simulink model "xmc_optical_flow"  (R2019b)
settings: Solver=VariableStepAuto  StartTime=0.0  StopTime=inf  RelTol=1e-3  EnableMultiTasking=on
PostLoadFcn:
  | xmcHubUpdateInstalledDevice(gcs);
model workspace (MAT data in the model file):
  SourceMovingObject = 0
  gainValueHSV = 0.2
undefined symbols (not defined in the file or in its folder): A, AXI4, gray, Kanade, Lucas, N, Rec, SDTV, Stream, xc7vx485tffg1157
libraries: ModelComposer x66, visionconversions x3, visiongeotforms x2, xmcCopyrightNotice x1, visionsinks x1, OpticalFlowRoots x1, visionsources x1, visionutilities x1, dspvision x1
settings Model: Creator=abehbood  LastModifiedBy=abehbood
settings DataIOCC: ReturnWorkspaceOutputs=off
settings OptimizationCC: EfficientMapNaN2IntZero=off  LifeSpan=inf
settings DebuggingCC: SFUnexpectedBacktrackingDiag=warning  SFNoUnconditionalDefaultTransitionDiag=warning  ArithmeticOperatorsInVariantConditions=warning
settings HardwareCC: TargetBitPerLong=64  TargetBitPerPointer=64  TargetBitPerSizeT=64  TargetBitPerPtrDiffT=64  TargetLongLongMode=on  TargetIntDivRoundTo=Zero  TargetEndianess=LittleEndian  TargetWordSize=64  TargetHWDeviceType=MATLAB Host  ProdEqTarget=off
settings SFSimCC: SimUseLocalCustomCode=off  CustomCodeUndefinedFunction=UseInterfaceOnly
settings RTWCC: RTWUseLocalCustomCode=off
settings CodeAppCC: MaxIdLength=128  StateflowObjectComments=on
settings GRTTargetCC: TargetLangStandard=C89/C90 (ANSI)  CombineOutputUpdateFcns=off  GRTInterface=on
settings ConfigComp: CovMetricSettings=dw  CovHtmlReporting=on  CovSaveCumulativeToWorkspaceVar=on  CovSaveSingleToWorkspaceVar=on  CovExternalEMLEnable=off

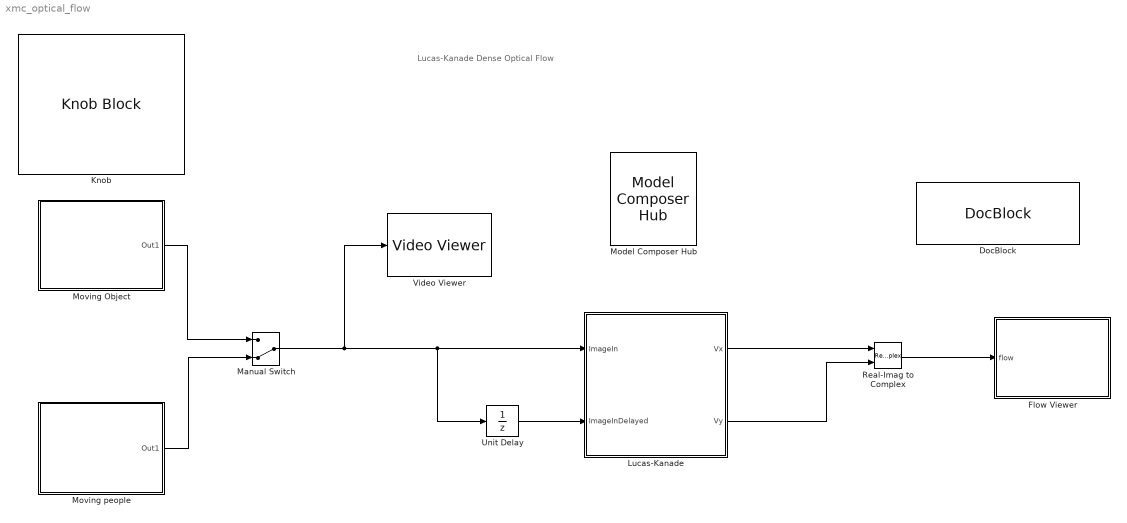
== system xmc_optical_flow ==
  note: Lucas-Kanade Dense Optical Flow
  DocBlock : xmcCopyrightNotice/DocBlock
      content=|
      | (c) Copyright 2017-2018 Xilinx, Inc. All rights reserved.
      |
      | This file contains confidential and proprietary information of Xilinx, Inc.
      | and is protected under U.S. and international copyright and other
      | intellectual property laws.
      |
      | DISCLAIMER
      | This disclaimer is not a license and does not grant any rights to the
      | materials distributed herewith. Except as otherwise provided in a valid
      | license issued to you by Xilinx, and to the maximum extent permitted by
      | applicable law: (1) THESE MATERIALS ARE MADE AVAILABLE "AS IS" AND WITH
      | ALL FAULTS, AND XILINX HEREBY DISCLAIMS ALL WARRANTIES AND CONDITIONS,
      | EXPRESS, IMPLIED, OR STATUTORY, INCLUDING BUT NOT LIMITED TO WARRANTIES
      | OF MERCHANTABILITY, NON-INFRINGEMENT, OR FITNESS FOR ANY PARTICULAR
      | PURPOSE; and (2) Xilinx shall not be liable (whether in contract or tort,
      | including negligence, or under any other theory of liability) for any
      | loss or damage of any kind or nature related to, arising under or in
      | connection with these materials, including for any direct, or any indirect,
      | special, incidental, or consequential loss or damage (including loss of
      | data, profits, goodwill, or any type of loss or damage suffered as a
      | result of any action brought by a third party) even if such damage or loss
      | was reasonably foreseeable or Xilinx had been advised of the possibility
      | of the same.
      |
      | CRITICAL APPLICATIONS
      | Xilinx products are not designed or intended to be fail-safe, or for use
      | in any application requiring fail-safe performance, such as life-support
      | or safety devices or systems, Class III medical devices, nuclear
      | facilities, applications related to the deployment of airbags, or
      | any other applications that could lead to death, personal injury, or
      | severe property or environmental damage (individually and collectively,
      | "Critical Applications"). Customer assumes the sole risk and liability
      | of any use of Xilinx products in Critical Applications, subject only to
      | applicable laws and regulations governing limitations on product liability.
      |
      | THIS COPYRIGHT NOTICE AND DISCLAIMER MUST BE RETAINED AS PART OF
      | THIS FILE AT ALL TIMES.
      settings: SourceProductName=Simulink  SourceProductBaseCode=SL
  Flow Viewer : Subsystem
  Knob : KnobBlock  ScaleMin=-180  ScaleMax=180  TickInterval=45
  Lucas-Kanade : Subsystem  mask{thresh=.0015, d5=[-1 8 0 -8 1]/12, p5=[1 4 6 4 1]/16, b=ones(1,5)/5}
      mask prompts: thresh "Threshold"; d5 "Gradient filter"; p5 "Smoothing filter"; b "Box filter"
      mask init:
      | K  = p5(:)*p5(:)';
  Manual Switch : ManualSwitch  CurrentSetting=0
      settings: OpenFcn=switchCallback(gcb)
  Model Composer Hub : ModelComposer/Model Composer Hub  CodeGeneration=off  SubsystemName=Lucas-Kanade  TargetDirectory=./code  ExportType=HLS C++ code  IpVendor=xilinx.com  IpLibrary=hls  IpVersion=1.0  IpHWLanguage=Verilog  AieCompilerOptions={}  CreateTestbench=off  TestbenchStackSize=10  RunAieSim=off  AieSimTimeout=50000  LaunchVitisAnalyzer=off  RunX86Sim=on  X86SimTimeout=10  ProjDevice=xc7vx485tffg1157-1  ProjDevicePart=xc7vx485tffg1157-1  SamplePeriod=-1  ClockFrequency=300  DataPathParallelism=1
  Moving Object : Subsystem  mask{Angle=98.39185180664066}
      mask prompts: Angle "Angle of motion in degrees:"
  Moving people : Subsystem
  Real-Imag to Complex : RealImagToComplex
  Unit Delay : UnitDelay  SampleTime=-1  HasFrameUpgradeWarning=on
  Video Viewer : VideoViewer  colormapValue=gray(256)  FigPos=[735 508 863 363]
  wires:
  Lucas-Kanade/1(Vx) -> Real-Imag to Complex/1
  Lucas-Kanade/2(Vy) -> Real-Imag to Complex/2
  Unit Delay/1 -> Lucas-Kanade/2(ImageInDelayed)
  Manual Switch/1 -> Unit Delay/1, Lucas-Kanade/1(ImageIn), Video Viewer/1
  Real-Imag to Complex/1 -> Flow Viewer/1(flow)
  Moving Object/1(Out1) -> Manual Switch/1
  Moving people/1(Out1) -> Manual Switch/2

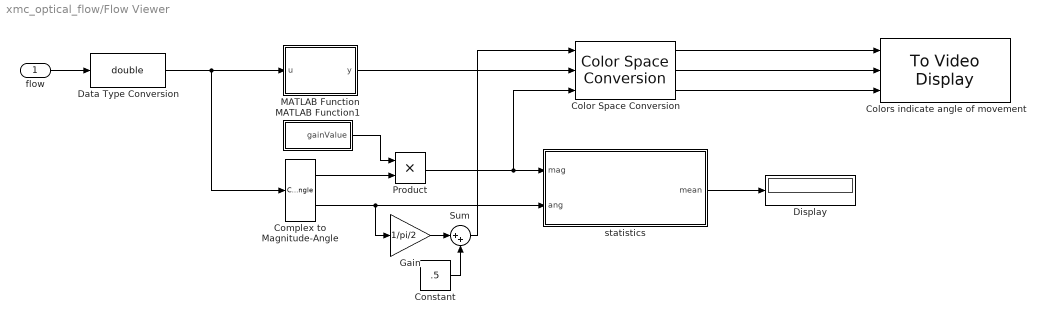
== system xmc_optical_flow/Flow Viewer ==
  flow : Inport
  Color Space Conversion : visionconversions/Color Space  Conversion  conversion=Obsolete  conversionActive=HSV to R'G'B'  wp_str=D65  rec=Rec. 601 (SDTV)  sys=1125/60/2:1  imagePorts=Separate color signals
  Colors indicate angle of movement : visionsinks/To Video Display  windowSizeMode=Normal  openAtMdlStart=on  fullScreen=off  videoWindowX=1226  videoWindowY=338  saveWindowSize=off  videoWindowWidth=670  videoWindowHeight=374  inputColorFormat=RGB  inputType=Obsolete  imagePorts=Separate color signals  OutputDevice=On-screen video monitor  dataOrg=Column-major  isWindowOpen=off
      settings: SourceProductName=Computer Vision Toolbox
  Complex to Magnitude-Angle : ComplexToMagnitudeAngle
  Constant : Constant  Value=.5
  Data Type Conversion : DataTypeConversion  OutDataTypeStr=double
  Display : Display
  Gain : Gain  Gain=1/pi/2  OutDataTypeStr=double
  MATLAB Function : MATLAB Function  TreatAsAtomicUnit=on
  MATLAB Function1 : MATLAB Function  TreatAsAtomicUnit=on
  Product : Product
  Sum : Sum  Inputs=|++
  statistics : MATLAB Function  TreatAsAtomicUnit=on
  wires:
  Color Space Conversion/3 -> Colors indicate angle of movement/3
  Color Space Conversion/2 -> Colors indicate angle of movement/2
  Color Space Conversion/1 -> Colors indicate angle of movement/1
  statistics/1(mean) -> Display/1
  Constant/1 -> Sum/2
  Sum/1 -> Color Space Conversion/1
  Gain/1 -> Sum/1
  Complex to Magnitude-Angle/1 -> Product/2
  MATLAB Function/1(y) -> Color Space Conversion/2
  Complex to Magnitude-Angle/2 -> Gain/1, statistics/2(ang)
  flow/1 -> Data Type Conversion/1
  Data Type Conversion/1 -> MATLAB Function/1(u), Complex to Magnitude-Angle/1
  Product/1 -> Color Space Conversion/3, statistics/1(mag)
  MATLAB Function1/1(gainValue) -> Product/1

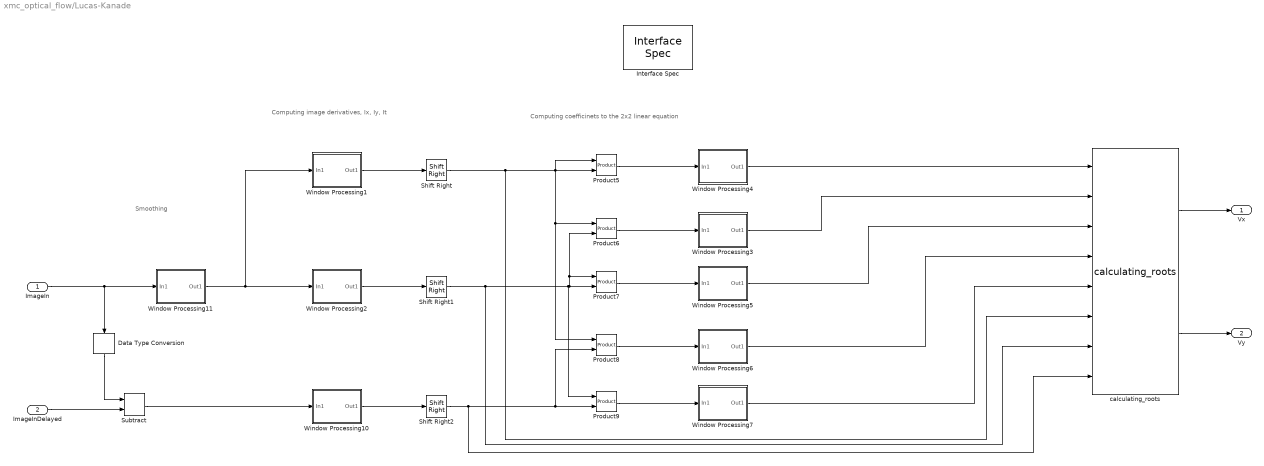
== system xmc_optical_flow/Lucas-Kanade ==
  note: Computing coefficinets to the 2x2
      |  linear equation
  note: Smoothing
  note: Computing image
      | derivatives, Ix, Iy, It
  ImageIn : Inport
  ImageInDelayed : Inport  Port=2
  Data Type Conversion : ModelComposer/Data Type Conversion  OutDataType=fixed  TypeExp=''  Signedness=Unsigned  WordLength=8  FractionalLength=0  RoundingMode=Truncation to minus infinity  OverflowMode=Wrap around
  Interface Spec : ModelComposer/Interface Spec  Return=AXI4-Lite Slave@@  InportInterfaces={'AXI4-Stream@@@N/A@N/A', 'AXI4-Stream@@@N/A@N/A'}  InportHandles={1.300039062500000000e+02, 1.310039062500000000e+02}  InportNames={'ImageIn', 'ImageInDelayed'}  OutportInterfaces={'AXI4-Stream@@@N/A@N/A', 'AXI4-Stream@@@N/A@N/A'}  OutportHandles={3.710037841796875000e+02, 3.720037841796875000e+02}  OutportNames={'Vx', 'Vy'}  Mode=AXI4-Lite Slave  InName1=In1  InMode1=AXI4-Stream  InVFormat1=N/A  InVComponent1=N/A  InName2=In2  InMode2=AXI4-Stream  InVFormat2=N/A  InVComponent2=N/A  InMode3=Default  InVFormat3=N/A  InVComponent3=N/A  InMode4=Default  InVFormat4=N/A  InVComponent4=N/A  InMode5=Default  InVFormat5=N/A  InVComponent5=N/A  InMode6=Default  InVFormat6=N/A  InVComponent6=N/A  InMode7=Default  InVFormat7=N/A  InVComponent7=N/A  InMode8=Default  InVFormat8=N/A  InVComponent8=N/A  OutName1=Out1  OutMode1=AXI4-Stream  OutVFormat1=N/A  OutVComponent1=N/A  OutName2=Out2  OutMode2=AXI4-Stream  OutVFormat2=N/A  OutVComponent2=N/A  OutMode3=Default  OutVFormat3=N/A  OutVComponent3=N/A  OutMode4=Default  OutVFormat4=N/A  OutVComponent4=N/A  OutMode5=Default  OutVFormat5=N/A  OutVComponent5=N/A  OutMode6=Default  OutVFormat6=N/A  OutVComponent6=N/A  OutMode7=Default  OutVFormat7=N/A  OutVComponent7=N/A  OutMode8=Default  OutVFormat8=N/A  OutVComponent8=N/A
  Product{5..9} (5 alike) : ModelComposer/Product
  Shift Right : ModelComposer/Shift Right  ShiftAmount=8
  Shift Right1 : ModelComposer/Shift Right  ShiftAmount=8
  Shift Right2 : ModelComposer/Shift Right  ShiftAmount=8
  Subtract : ModelComposer/Subtract
  Window Processing1 : Subsystem  mask(Window Processing){WindowSize=[1, 5], OutputSize=Same as Input}
      mask prompts: WindowSize "Window Size"; OutputSize "Output Size"
      mask help: Assembles output matrix by applying the kernel subsystem to sub matrices (windows) of the input matrix in row-major order.
      mask init:
      | set_param(gcb, 'LinkStatus', 'inactive');
      mask Help: helpview([xmcGetBlockHTMLPath 'windowprocessing.html']);
      mask TypeOptions WindowSize:
      | Window Processing
      | Master/WindowSize
      mask TypeOptions OutputSize:
      | Window Processing
      | Master/OutputSize
      mask DialogControl Container1 Prompt: Parameters
      mask DialogControl Control5 Prompt: Open Subsystem
      mask DialogControl Control5 Callback:
      | gcb
      | open_system([gcb , '/Kernel'])
      mask Display:
      | xmcDrawBlockIcon();
      | disp('\fontsize{10}   Window \newlineProcessing','texmode','on');
  Window Processing10 : Subsystem  mask(Window Processing){WindowSize=[5, 5], OutputSize=Same as Input}
      mask prompts: WindowSize "Window Size"; OutputSize "Output Size"
      mask help: Assembles output matrix by applying the kernel subsystem to sub matrices (windows) of the input matrix in row-major order.
      mask init:
      | set_param(gcb, 'LinkStatus', 'inactive');
      mask Help: helpview([xmcGetBlockHTMLPath 'windowprocessing.html']);
      mask TypeOptions WindowSize:
      | Window Processing
      | Master/WindowSize
      mask TypeOptions OutputSize:
      | Window Processing
      | Master/OutputSize
      mask DialogControl Container1 Prompt: Parameters
      mask DialogControl Control5 Prompt: Open Subsystem
      mask DialogControl Control5 Callback:
      | gcb
      | open_system([gcb , '/Kernel'])
      mask Display:
      | xmcDrawBlockIcon();
      | disp('\fontsize{10}   Window \newlineProcessing','texmode','on');
  Window Processing11 : Subsystem  mask(Window Processing){WindowSize=[5, 5], OutputSize=Same as Input}
      mask prompts: WindowSize "Window Size"; OutputSize "Output Size"
      mask help: Assembles output matrix by applying the kernel subsystem to sub matrices (windows) of the input matrix in row-major order.
      mask init:
      | set_param(gcb, 'LinkStatus', 'inactive');
      mask Help: helpview([xmcGetBlockHTMLPath 'windowprocessing.html']);
      mask TypeOptions WindowSize:
      | Window Processing
      | Master/WindowSize
      mask TypeOptions OutputSize:
      | Window Processing
      | Master/OutputSize
      mask DialogControl Container1 Prompt: Parameters
      mask DialogControl Control5 Prompt: Open Subsystem
      mask DialogControl Control5 Callback:
      | gcb
      | open_system([gcb , '/Kernel'])
      mask Display:
      | xmcDrawBlockIcon();
      | disp('\fontsize{10}   Window \newlineProcessing','texmode','on');
  Window Processing2 : Subsystem  mask(Window Processing){WindowSize=[5,1], OutputSize=Same as Input}
      mask prompts: WindowSize "Window Size"; OutputSize "Output Size"
      mask help: Assembles output matrix by applying the kernel subsystem to sub matrices (windows) of the input matrix in row-major order.
      mask init:
      | set_param(gcb, 'LinkStatus', 'inactive');
      mask Help: helpview([xmcGetBlockHTMLPath 'windowprocessing.html']);
      mask TypeOptions WindowSize:
      | Window Processing
      | Master/WindowSize
      mask TypeOptions OutputSize:
      | Window Processing
      | Master/OutputSize
      mask DialogControl Container1 Prompt: Parameters
      mask DialogControl Control5 Prompt: Open Subsystem
      mask DialogControl Control5 Callback:
      | gcb
      | open_system([gcb , '/Kernel'])
      mask Display:
      | xmcDrawBlockIcon();
      | disp('\fontsize{10}   Window \newlineProcessing','texmode','on');
  Window Processing3 : Subsystem  mask(Window Processing){WindowSize=[5,5], OutputSize=Same as Input}
      mask prompts: WindowSize "Window Size"; OutputSize "Output Size"
      mask help: Assembles output matrix by applying the kernel subsystem to sub matrices (windows) of the input matrix in row-major order.
      mask init:
      | set_param(gcb, 'LinkStatus', 'inactive');
      mask Help: helpview([xmcGetBlockHTMLPath 'windowprocessing.html']);
      mask TypeOptions WindowSize:
      | Window Processing
      | Master/WindowSize
      mask TypeOptions OutputSize:
      | Window Processing
      | Master/OutputSize
      mask DialogControl Container1 Prompt: Parameters
      mask DialogControl Control5 Prompt: Open Subsystem
      mask DialogControl Control5 Callback:
      | gcb
      | open_system([gcb , '/Kernel'])
      mask Display:
      | xmcDrawBlockIcon();
      | disp('\fontsize{10}   Window \newlineProcessing','texmode','on');
  Window Processing4 : Subsystem  mask(Window Processing){WindowSize=[5,5], OutputSize=Same as Input}
      mask prompts: WindowSize "Window Size"; OutputSize "Output Size"
      mask help: Assembles output matrix by applying the kernel subsystem to sub matrices (windows) of the input matrix in row-major order.
      mask init:
      | set_param(gcb, 'LinkStatus', 'inactive');
      mask Help: helpview([xmcGetBlockHTMLPath 'windowprocessing.html']);
      mask TypeOptions WindowSize:
      | Window Processing
      | Master/WindowSize
      mask TypeOptions OutputSize:
      | Window Processing
      | Master/OutputSize
      mask DialogControl Container1 Prompt: Parameters
      mask DialogControl Control5 Prompt: Open Subsystem
      mask DialogControl Control5 Callback:
      | gcb
      | open_system([gcb , '/Kernel'])
      mask Display:
      | xmcDrawBlockIcon();
      | disp('\fontsize{10}   Window \newlineProcessing','texmode','on');
  Window Processing5 : Subsystem  mask(Window Processing){WindowSize=[5,5], OutputSize=Same as Input}
      mask prompts: WindowSize "Window Size"; OutputSize "Output Size"
      mask help: Assembles output matrix by applying the kernel subsystem to sub matrices (windows) of the input matrix in row-major order.
      mask init:
      | set_param(gcb, 'LinkStatus', 'inactive');
      mask Help: helpview([xmcGetBlockHTMLPath 'windowprocessing.html']);
      mask TypeOptions WindowSize:
      | Window Processing
      | Master/WindowSize
      mask TypeOptions OutputSize:
      | Window Processing
      | Master/OutputSize
      mask DialogControl Container1 Prompt: Parameters
      mask DialogControl Control5 Prompt: Open Subsystem
      mask DialogControl Control5 Callback:
      | gcb
      | open_system([gcb , '/Kernel'])
      mask Display:
      | xmcDrawBlockIcon();
      | disp('\fontsize{10}   Window \newlineProcessing','texmode','on');
  Window Processing6 : Subsystem  mask(Window Processing){WindowSize=[5,5], OutputSize=Same as Input}
      mask prompts: WindowSize "Window Size"; OutputSize "Output Size"
      mask help: Assembles output matrix by applying the kernel subsystem to sub matrices (windows) of the input matrix in row-major order.
      mask init:
      | set_param(gcb, 'LinkStatus', 'inactive');
      mask Help: helpview([xmcGetBlockHTMLPath 'windowprocessing.html']);
      mask TypeOptions WindowSize:
      | Window Processing
      | Master/WindowSize
      mask TypeOptions OutputSize:
      | Window Processing
      | Master/OutputSize
      mask DialogControl Container1 Prompt: Parameters
      mask DialogControl Control5 Prompt: Open Subsystem
      mask DialogControl Control5 Callback:
      | gcb
      | open_system([gcb , '/Kernel'])
      mask Display:
      | xmcDrawBlockIcon();
      | disp('\fontsize{10}   Window \newlineProcessing','texmode','on');
  Window Processing7 : Subsystem  mask(Window Processing){WindowSize=[5,5], OutputSize=Same as Input}
      mask prompts: WindowSize "Window Size"; OutputSize "Output Size"
      mask help: Assembles output matrix by applying the kernel subsystem to sub matrices (windows) of the input matrix in row-major order.
      mask init:
      | set_param(gcb, 'LinkStatus', 'inactive');
      mask Help: helpview([xmcGetBlockHTMLPath 'windowprocessing.html']);
      mask TypeOptions WindowSize:
      | Window Processing
      | Master/WindowSize
      mask TypeOptions OutputSize:
      | Window Processing
      | Master/OutputSize
      mask DialogControl Container1 Prompt: Parameters
      mask DialogControl Control5 Prompt: Open Subsystem
      mask DialogControl Control5 Callback:
      | gcb
      | open_system([gcb , '/Kernel'])
      mask Display:
      | xmcDrawBlockIcon();
      | disp('\fontsize{10}   Window \newlineProcessing','texmode','on');
  calculating_roots : OpticalFlowRoots/calculating_roots  LibraryFunction=calculating_roots  IncludeFiles={'calculating_roots.h'}  SourceFiles={}  IncludeDirectories={}  TemplateParams={' '}  FunctionParamTypes={xmcDataType('void'); xmcDataType('int16_t'); xmcDataType('int16_t'); xmcDataType('int16_t'); xmcDataType('int16_t'); xmcDataType('int16_t'); xmcDataType('int16_t'); xmcDataType('int16_t'); xmcDataType('int16_t'); xmcDataType('float &'); xmcDataType('float &')}  FunctionParamPassbys={0.000000000000000000e+00; 0.000000000000000000e+00; 0.000000000000000000e+00; 0.000000000000000000e+00; 0.000000000000000000e+00; 0.000000000000000000e+00; 0.000000000000000000e+00; 0.000000000000000000e+00; 0.000000000000000000e+00; 1.000000000000000000e+00; 1.000000000000000000e+00}  FunctionParamDimensions={'1'; '1'; '1'; '1'; '1'; '1'; '1'; '1'; '1'; '1'; '1'}  FunctionParamNames={'return'; 'aPix'; 'bPix'; 'cPix'; 'txPix'; 'tyPix'; 'IxPix'; 'IyPix'; 'dtPix'; 'VxPix'; 'VyPix'}  FunctionParamDir={0.000000000000000000e+00; 1.000000000000000000e+00; 1.000000000000000000e+00; 1.000000000000000000e+00; 1.000000000000000000e+00; 1.000000000000000000e+00; 1.000000000000000000e+00; 1.000000000000000000e+00; 1.000000000000000000e+00; 2.000000000000000000e+00; 2.000000000000000000e+00}  FunctionParamSupportsStreaming={false; false; false; false; false; false; false; false; false; false; false}  BufferDepth={'0'}  FunctionParamValues={'0'; '0'; '0'; '0'; '0'; '0'; '0'; '0'; '0'; '0'; '0'}  ThroughputFactors={''}
  Vx : Outport
  Vy : Outport  Port=2
  wires:
  calculating_roots/1 -> Vx/1
  ImageIn/1 -> Data Type Conversion/1, Window Processing11/1(In1)
  Window Processing2/1(Out1) -> Shift Right1/1
  calculating_roots/2 -> Vy/1
  Window Processing10/1(Out1) -> Shift Right2/1
  ImageInDelayed/1 -> Subtract/2
  Window Processing11/1(Out1) -> Window Processing2/1(In1), Window Processing1/1(In1)
  Data Type Conversion/1 -> Subtract/1
  Subtract/1 -> Window Processing10/1(In1)
  Product5/1 -> Window Processing4/1(In1)
  Product6/1 -> Window Processing3/1(In1)
  Product8/1 -> Window Processing6/1(In1)
  Product7/1 -> Window Processing5/1(In1)
  Product9/1 -> Window Processing7/1(In1)
  Shift Right2/1 -> calculating_roots/8, Product9/2, Product8/2
  Window Processing4/1(Out1) -> calculating_roots/1
  Window Processing3/1(Out1) -> calculating_roots/2
  Window Processing5/1(Out1) -> calculating_roots/3
  Window Processing6/1(Out1) -> calculating_roots/4
  Window Processing7/1(Out1) -> calculating_roots/5
  Shift Right/1 -> calculating_roots/6, Product5/1, Product5/2, Product6/1, Product8/1
  Shift Right1/1 -> calculating_roots/7, Product7/2, Product6/2, Product7/1, Product9/1
  Window Processing1/1(Out1) -> Shift Right/1

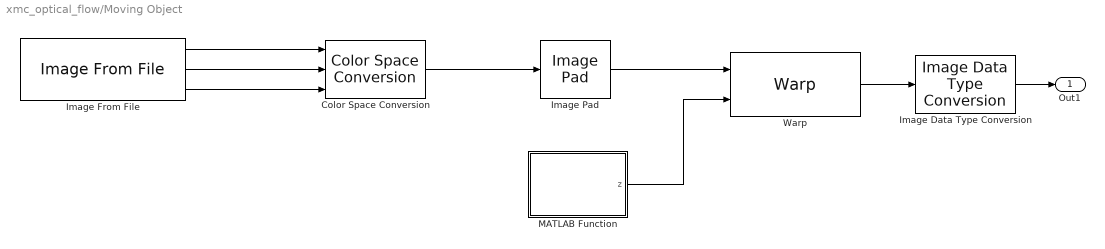
== system xmc_optical_flow/Moving Object ==
  Color Space Conversion : visionconversions/Color Space  Conversion  conversion=Obsolete  conversionActive=R'G'B' to intensity  wp_str=D65  rec=Rec. 601 (SDTV)  sys=1125/60/2:1  imagePorts=Separate color signals
  Image Data Type Conversion : visionconversions/Image Data Type Conversion  outDT=uint8  isSigned=on  wordLen=16  numFracBits=0
      settings: SourceProductName=Computer Vision Toolbox  SourceProductBaseCode=VP
  Image From File : visionsources/Image From File  Tag=vipblks_nd  FileName=object.png  Ts=1  imagePorts=Separate color signals  OutPortLabels=R|G|B  ImageDataType=double  sdImageDataType=uint(8)  Signed=on  WordLength=16  FractionLengthMode=User-defined  FractionLength=15
      settings: SourceProductName=Computer Vision Toolbox
  Image Pad : visionutilities/Image Pad  method=Constant  valSrc=Specify via dialog  value=0  spec=Pad size  rowDirection=Both left and right  outRowsMode=User-specified  rowSize=95  outColSize=10  colDirection=Both top and bottom  outColsMode=User-specified  colSize=95  outRowSize=12  trunc_flag=None
      settings: SourceProductName=Computer Vision Toolbox  SourceProductBaseCode=VP
  MATLAB Function : MATLAB Function  TreatAsAtomicUnit=on
  Warp : visiongeotforms/Warp  TransformMatrixSource=Input port  TransformMatrix=eye( 3 )  InterpolationMethod=Bilinear  BackgroundFillValue=0  OutputImagePositionSource=Same as input image  OutputImagePosition=[ 1, 1, 512, 512 ]  ROIInputPort=off  ROIValidityOutputPort=off  SimulateUsing=Interpreted execution
      settings: SourceProductName=Computer Vision Toolbox  SourceProductBaseCode=VP
  Out1 : Outport
  wires:
  Image Data Type Conversion/1 -> Out1/1
  Color Space Conversion/1 -> Image Pad/1
  Image From File/3 -> Color Space Conversion/3
  Image Pad/1 -> Warp/1
  Image From File/1 -> Color Space Conversion/1
  Image From File/2 -> Color Space Conversion/2
  MATLAB Function/1(z) -> Warp/2
  Warp/1 -> Image Data Type Conversion/1

== system xmc_optical_flow/Moving people ==
  From Multimedia File : dspvision/From Multimedia File  inputFilename=vipmen.avi  readRange=[1 Inf]  loop=on  numPlays=inf  outputStreams=Video only  videoDataType=uint8  audioDataType=int16  inheritSampleTime=off  userDefinedSampleTime=1  noAudioOutput=off  isIntensityVideo=off  fourcc=Intensity  colorVideoFormat=One multidimensional signal  outputEOF=off  dataOrg=Column-major  audioFrameSize=1024  computeAudioFrameSize=off  outSamplingMode=Sample based
      settings: SourceProductName=DSP System Toolbox  SourceProductBaseCode=DS
  Resize : visiongeotforms/Resize  specify=Number of output rows and columns  rfactor=[200 150]  outCols=25  outRows=25  outRowsCols=[200 200]  interp_method=Bilinear  antialias=on  useROI=off  roiFlag=off  roundingMode=Nearest  overflowMode=on  prodOutputMode=Binary point scaling  prodOutputWordLength=32  prodOutputFracLength=10  prodOutputSlope=2^-10  accumSlope=2^-10  outputSlope=2^-10
      settings: SourceProductName=Computer Vision Toolbox  SourceProductBaseCode=VP
  Out1 : Outport
  wires:
  Resize/1 -> Out1/1
  From Multimedia File/1 -> Resize/1

== system xmc_optical_flow/Lucas-Kanade/Window Processing1 ==
  In1 : Inport
  Kernel : Subsystem
  Window Processing Master : ModelComposer/Window Processing Master  Description=Performs multiplication  WindowSize=WindowSize  OutputSize=Same as Input
  Window Processing Slave : ModelComposer/Window Processing Slave  Description=Performs multiplication
  Out1 : Outport
  wires:
  Window Processing Slave/1 -> Window Processing Master/2
  Kernel/1(Out1) -> Window Processing Slave/1
  Window Processing Master/2 -> Kernel/1(In1)
  In1/1 -> Window Processing Master/1
  Window Processing Master/1 -> Out1/1

== system xmc_optical_flow/Lucas-Kanade/Window Processing10 ==
  In1 : Inport
  Kernel : Subsystem
  Window Processing Master : ModelComposer/Window Processing Master  Description=Performs multiplication  WindowSize=WindowSize  OutputSize=Same as Input
  Window Processing Slave : ModelComposer/Window Processing Slave  Description=Performs multiplication
  Out1 : Outport
  wires:
  Window Processing Slave/1 -> Window Processing Master/2
  Kernel/1(Out1) -> Window Processing Slave/1
  Window Processing Master/2 -> Kernel/1(In1)
  In1/1 -> Window Processing Master/1
  Window Processing Master/1 -> Out1/1

== system xmc_optical_flow/Lucas-Kanade/Window Processing11 ==
  In1 : Inport
  Kernel : Subsystem
  Window Processing Master : ModelComposer/Window Processing Master  Description=Performs multiplication  WindowSize=WindowSize  OutputSize=Same as Input
  Window Processing Slave : ModelComposer/Window Processing Slave  Description=Performs multiplication
  Out1 : Outport
  wires:
  Window Processing Master/1 -> Out1/1
  In1/1 -> Window Processing Master/1
  Window Processing Master/2 -> Kernel/1(In1)
  Kernel/1(Out1) -> Window Processing Slave/1
  Window Processing Slave/1 -> Window Processing Master/2

== system xmc_optical_flow/Lucas-Kanade/Window Processing2 ==
  In1 : Inport
  Kernel : Subsystem
  Window Processing Master : ModelComposer/Window Processing Master  Description=Performs multiplication  WindowSize=WindowSize  OutputSize=Same as Input
  Window Processing Slave : ModelComposer/Window Processing Slave  Description=Performs multiplication
  Out1 : Outport
  wires:
  Window Processing Master/1 -> Out1/1
  In1/1 -> Window Processing Master/1
  Window Processing Master/2 -> Kernel/1(In1)
  Kernel/1(Out1) -> Window Processing Slave/1
  Window Processing Slave/1 -> Window Processing Master/2

== system xmc_optical_flow/Lucas-Kanade/Window Processing3 ==
  In1 : Inport
  Kernel : Subsystem
  Window Processing Master : ModelComposer/Window Processing Master  Description=Performs multiplication  WindowSize=WindowSize  OutputSize=Same as Input
  Window Processing Slave : ModelComposer/Window Processing Slave  Description=Performs multiplication
  Out1 : Outport
  wires:
  Window Processing Slave/1 -> Window Processing Master/2
  Kernel/1(Out1) -> Window Processing Slave/1
  Window Processing Master/2 -> Kernel/1(In1)
  In1/1 -> Window Processing Master/1
  Window Processing Master/1 -> Out1/1

== system xmc_optical_flow/Lucas-Kanade/Window Processing4 ==
  In1 : Inport
  Kernel : Subsystem
  Window Processing Master : ModelComposer/Window Processing Master  Description=Performs multiplication  WindowSize=WindowSize  OutputSize=Same as Input
  Window Processing Slave : ModelComposer/Window Processing Slave  Description=Performs multiplication
  Out1 : Outport
  wires:
  Window Processing Master/1 -> Out1/1
  In1/1 -> Window Processing Master/1
  Window Processing Master/2 -> Kernel/1(In1)
  Kernel/1(Out1) -> Window Processing Slave/1
  Window Processing Slave/1 -> Window Processing Master/2

== system xmc_optical_flow/Lucas-Kanade/Window Processing5 ==
  In1 : Inport
  Kernel : Subsystem
  Window Processing Master : ModelComposer/Window Processing Master  Description=Performs multiplication  WindowSize=WindowSize  OutputSize=Same as Input
  Window Processing Slave : ModelComposer/Window Processing Slave  Description=Performs multiplication
  Out1 : Outport
  wires:
  Window Processing Master/1 -> Out1/1
  In1/1 -> Window Processing Master/1
  Window Processing Master/2 -> Kernel/1(In1)
  Kernel/1(Out1) -> Window Processing Slave/1
  Window Processing Slave/1 -> Window Processing Master/2

== system xmc_optical_flow/Lucas-Kanade/Window Processing6 ==
  In1 : Inport
  Kernel : Subsystem
  Window Processing Master : ModelComposer/Window Processing Master  Description=Performs multiplication  WindowSize=WindowSize  OutputSize=Same as Input
  Window Processing Slave : ModelComposer/Window Processing Slave  Description=Performs multiplication
  Out1 : Outport
  wires:
  Window Processing Slave/1 -> Window Processing Master/2
  Kernel/1(Out1) -> Window Processing Slave/1
  Window Processing Master/2 -> Kernel/1(In1)
  In1/1 -> Window Processing Master/1
  Window Processing Master/1 -> Out1/1

== system xmc_optical_flow/Lucas-Kanade/Window Processing7 ==
  In1 : Inport
  Kernel : Subsystem
  Window Processing Master : ModelComposer/Window Processing Master  Description=Performs multiplication  WindowSize=WindowSize  OutputSize=Same as Input
  Window Processing Slave : ModelComposer/Window Processing Slave  Description=Performs multiplication
  Out1 : Outport
  wires:
  Window Processing Master/1 -> Out1/1
  In1/1 -> Window Processing Master/1
  Window Processing Master/2 -> Kernel/1(In1)
  Kernel/1(Out1) -> Window Processing Slave/1
  Window Processing Slave/1 -> Window Processing Master/2

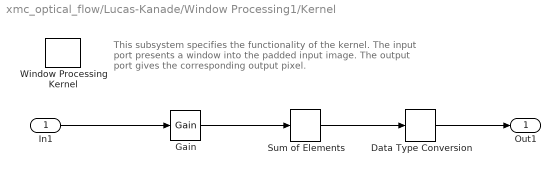
== system xmc_optical_flow/Lucas-Kanade/Window Processing1/Kernel ==
  note: This subsystem specifies the functionality of the kernel.
      | The input port presents a window into the padded input image.
      | The output port gives the corresponding output pixel.
  In1 : Inport
  Data Type Conversion : ModelComposer/Data Type Conversion  OutDataType=int16  TypeExp=''  Signedness=Signed  WordLength=16  FractionalLength=0  RoundingMode=Truncation to minus infinity  OverflowMode=Wrap around
  Gain : ModelComposer/Gain  Gain=fliplr(d5(:)')*256  OutDataType=fixed  TypeExp=''  Signedness=Signed  WordLength=9  FractionalLength=0  RoundingMode=Truncation to minus infinity  OverflowMode=Wrap around  OutputTypeAsInput=off
  Sum of Elements : ModelComposer/Sum of Elements  CollapseDim=2
  Window Processing Kernel : ModelComposer/Window Processing Kernel  Description=Performs multiplication  SubsystemName='optical_flow_moc/Lucas-Kanade/Window Processing1/Kernel'  TargetDirectory='./Kernel'
  Out1 : Outport
  wires:
  In1/1 -> Gain/1
  Gain/1 -> Sum of Elements/1
  Sum of Elements/1 -> Data Type Conversion/1
  Data Type Conversion/1 -> Out1/1

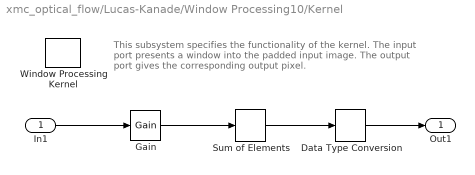
== system xmc_optical_flow/Lucas-Kanade/Window Processing10/Kernel ==
  note: This subsystem specifies the functionality of the kernel.
      | The input port presents a window into the padded input image.
      | The output port gives the corresponding output pixel.
  In1 : Inport
  Data Type Conversion : ModelComposer/Data Type Conversion  OutDataType=int16  TypeExp=''  Signedness=Signed  WordLength=16  FractionalLength=0  RoundingMode=Truncation to minus infinity  OverflowMode=Wrap around
  Gain : ModelComposer/Gain  Gain=p5(:)*p5(:)'*256  OutDataType=uint8  TypeExp=''  Signedness=Unsigned  WordLength=16  FractionalLength=16  RoundingMode=Truncation to minus infinity  OverflowMode=Wrap around  OutputTypeAsInput=off
  Sum of Elements : ModelComposer/Sum of Elements  CollapseDim=1
  Window Processing Kernel : ModelComposer/Window Processing Kernel  Description=Performs multiplication  SubsystemName='optical_flow_moc/Lucas-Kanade/Window Processing/Kernel'  TargetDirectory='./Kernel'
  Out1 : Outport
  wires:
  In1/1 -> Gain/1
  Gain/1 -> Sum of Elements/1
  Sum of Elements/1 -> Data Type Conversion/1
  Data Type Conversion/1 -> Out1/1

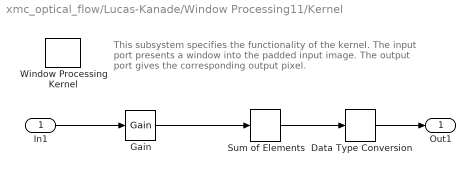
== system xmc_optical_flow/Lucas-Kanade/Window Processing11/Kernel ==
  note: This subsystem specifies the functionality of the kernel.
      | The input port presents a window into the padded input image.
      | The output port gives the corresponding output pixel.
  In1 : Inport
  Data Type Conversion : ModelComposer/Data Type Conversion  OutDataType=uint8  TypeExp=''  Signedness=Signed  WordLength=9  FractionalLength=0  RoundingMode=Truncation to minus infinity  OverflowMode=Wrap around
  Gain : ModelComposer/Gain  Gain=p5(:)*p5(:)'  OutDataType=fixed  TypeExp=''  Signedness=Unsigned  WordLength=16  FractionalLength=16  RoundingMode=Truncation to minus infinity  OverflowMode=Wrap around  OutputTypeAsInput=off
  Sum of Elements : ModelComposer/Sum of Elements  CollapseDim=1
  Window Processing Kernel : ModelComposer/Window Processing Kernel  Description=Performs multiplication  SubsystemName='optical_flow_moc/Lucas-Kanade/Window Processing/Kernel'  TargetDirectory='./Kernel'
  Out1 : Outport
  wires:
  Data Type Conversion/1 -> Out1/1
  Sum of Elements/1 -> Data Type Conversion/1
  Gain/1 -> Sum of Elements/1
  In1/1 -> Gain/1

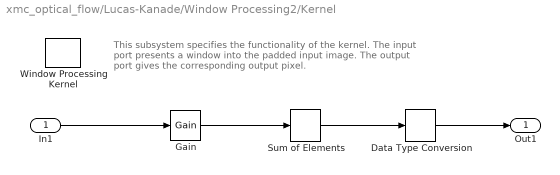
== system xmc_optical_flow/Lucas-Kanade/Window Processing2/Kernel ==
  note: This subsystem specifies the functionality of the kernel.
      | The input port presents a window into the padded input image.
      | The output port gives the corresponding output pixel.
  In1 : Inport
  Data Type Conversion : ModelComposer/Data Type Conversion  OutDataType=int16  TypeExp=''  Signedness=Signed  WordLength=16  FractionalLength=0  RoundingMode=Truncation to minus infinity  OverflowMode=Wrap around
  Gain : ModelComposer/Gain  Gain=flipud(d5(:))*256  OutDataType=fixed  TypeExp=''  Signedness=Signed  WordLength=9  FractionalLength=0  RoundingMode=Truncation to minus infinity  OverflowMode=Wrap around  OutputTypeAsInput=off
  Sum of Elements : ModelComposer/Sum of Elements  CollapseDim=2
  Window Processing Kernel : ModelComposer/Window Processing Kernel  Description=Performs multiplication  SubsystemName='optical_flow_moc/Lucas-Kanade/Window Processing1/Kernel'  TargetDirectory='./Kernel'
  Out1 : Outport
  wires:
  Data Type Conversion/1 -> Out1/1
  Sum of Elements/1 -> Data Type Conversion/1
  Gain/1 -> Sum of Elements/1
  In1/1 -> Gain/1

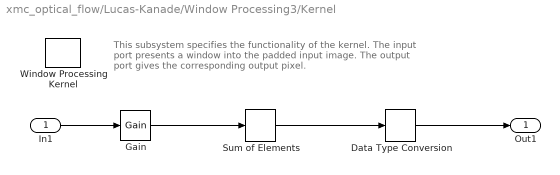
== system xmc_optical_flow/Lucas-Kanade/Window Processing3/Kernel ==
  note: This subsystem specifies the functionality of the kernel.
      | The input port presents a window into the padded input image.
      | The output port gives the corresponding output pixel.
  In1 : Inport
  Data Type Conversion : ModelComposer/Data Type Conversion  OutDataType=int16  TypeExp=''  Signedness=Signed  WordLength=16  FractionalLength=0  RoundingMode=Truncation to minus infinity  OverflowMode=Wrap around
  Gain : ModelComposer/Gain  Gain=1/25  OutDataType=fixed  TypeExp=''  Signedness=Unsigned  WordLength=10  FractionalLength=10  RoundingMode=Truncation to minus infinity  OverflowMode=Wrap around  OutputTypeAsInput=off
  Sum of Elements : ModelComposer/Sum of Elements  CollapseDim=2
  Window Processing Kernel : ModelComposer/Window Processing Kernel  Description=Performs multiplication  SubsystemName='optical_flow_moc/Lucas-Kanade/Window Processing1/Kernel'  TargetDirectory='./Kernel'
  Out1 : Outport
  wires:
  In1/1 -> Gain/1
  Sum of Elements/1 -> Data Type Conversion/1
  Data Type Conversion/1 -> Out1/1
  Gain/1 -> Sum of Elements/1

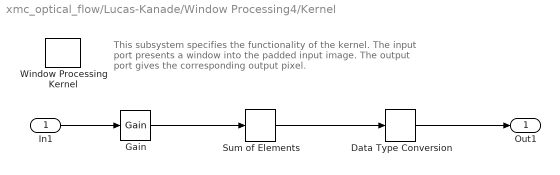
== system xmc_optical_flow/Lucas-Kanade/Window Processing4/Kernel ==
  note: This subsystem specifies the functionality of the kernel.
      | The input port presents a window into the padded input image.
      | The output port gives the corresponding output pixel.
  In1 : Inport
  Data Type Conversion : ModelComposer/Data Type Conversion  OutDataType=int16  TypeExp=''  Signedness=Signed  WordLength=16  FractionalLength=0  RoundingMode=Truncation to minus infinity  OverflowMode=Wrap around
  Gain : ModelComposer/Gain  Gain=1/25  OutDataType=fixed  TypeExp=''  Signedness=Unsigned  WordLength=10  FractionalLength=10  RoundingMode=Truncation to minus infinity  OverflowMode=Wrap around  OutputTypeAsInput=off
  Sum of Elements : ModelComposer/Sum of Elements  CollapseDim=2
  Window Processing Kernel : ModelComposer/Window Processing Kernel  Description=Performs multiplication  SubsystemName='optical_flow_moc/Lucas-Kanade/Window Processing1/Kernel'  TargetDirectory='./Kernel'
  Out1 : Outport
  wires:
  Gain/1 -> Sum of Elements/1
  Data Type Conversion/1 -> Out1/1
  Sum of Elements/1 -> Data Type Conversion/1
  In1/1 -> Gain/1

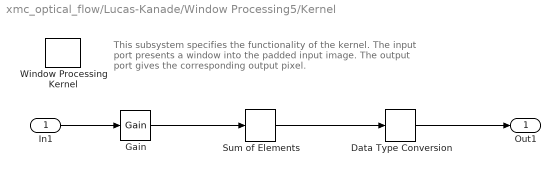
== system xmc_optical_flow/Lucas-Kanade/Window Processing5/Kernel ==
  note: This subsystem specifies the functionality of the kernel.
      | The input port presents a window into the padded input image.
      | The output port gives the corresponding output pixel.
  In1 : Inport
  Data Type Conversion : ModelComposer/Data Type Conversion  OutDataType=int16  TypeExp=''  Signedness=Signed  WordLength=16  FractionalLength=0  RoundingMode=Truncation to minus infinity  OverflowMode=Wrap around
  Gain : ModelComposer/Gain  Gain=1/25  OutDataType=fixed  TypeExp=''  Signedness=Unsigned  WordLength=10  FractionalLength=10  RoundingMode=Truncation to minus infinity  OverflowMode=Wrap around  OutputTypeAsInput=off
  Sum of Elements : ModelComposer/Sum of Elements  CollapseDim=2
  Window Processing Kernel : ModelComposer/Window Processing Kernel  Description=Performs multiplication  SubsystemName='optical_flow_moc/Lucas-Kanade/Window Processing1/Kernel'  TargetDirectory='./Kernel'
  Out1 : Outport
  wires:
  Gain/1 -> Sum of Elements/1
  Data Type Conversion/1 -> Out1/1
  Sum of Elements/1 -> Data Type Conversion/1
  In1/1 -> Gain/1

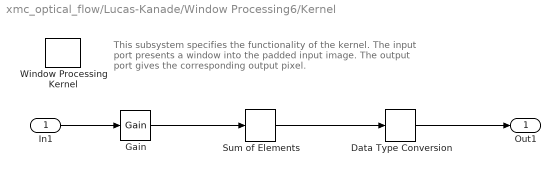
== system xmc_optical_flow/Lucas-Kanade/Window Processing6/Kernel ==
  note: This subsystem specifies the functionality of the kernel.
      | The input port presents a window into the padded input image.
      | The output port gives the corresponding output pixel.
  In1 : Inport
  Data Type Conversion : ModelComposer/Data Type Conversion  OutDataType=int16  TypeExp=''  Signedness=Signed  WordLength=16  FractionalLength=0  RoundingMode=Truncation to minus infinity  OverflowMode=Wrap around
  Gain : ModelComposer/Gain  Gain=1/25  OutDataType=fixed  TypeExp=''  Signedness=Unsigned  WordLength=10  FractionalLength=10  RoundingMode=Truncation to minus infinity  OverflowMode=Wrap around  OutputTypeAsInput=off
  Sum of Elements : ModelComposer/Sum of Elements  CollapseDim=2
  Window Processing Kernel : ModelComposer/Window Processing Kernel  Description=Performs multiplication  SubsystemName='optical_flow_moc/Lucas-Kanade/Window Processing1/Kernel'  TargetDirectory='./Kernel'
  Out1 : Outport
  wires:
  In1/1 -> Gain/1
  Sum of Elements/1 -> Data Type Conversion/1
  Data Type Conversion/1 -> Out1/1
  Gain/1 -> Sum of Elements/1

== system xmc_optical_flow/Lucas-Kanade/Window Processing7/Kernel ==
  note: This subsystem specifies the functionality of the kernel.
      | The input port presents a window into the padded input image.
      | The output port gives the corresponding output pixel.
  In1 : Inport
  Data Type Conversion : ModelComposer/Data Type Conversion  OutDataType=int16  TypeExp=''  Signedness=Signed  WordLength=16  FractionalLength=0  RoundingMode=Truncation to minus infinity  OverflowMode=Wrap around
  Gain : ModelComposer/Gain  Gain=1/25  OutDataType=fixed  TypeExp=''  Signedness=Unsigned  WordLength=10  FractionalLength=10  RoundingMode=Truncation to minus infinity  OverflowMode=Wrap around  OutputTypeAsInput=off
  Sum of Elements : ModelComposer/Sum of Elements  CollapseDim=2
  Window Processing Kernel : ModelComposer/Window Processing Kernel  Description=Performs multiplication  SubsystemName='optical_flow_moc/Lucas-Kanade/Window Processing1/Kernel'  TargetDirectory='./Kernel'
  Out1 : Outport
  wires:
  Gain/1 -> Sum of Elements/1
  Data Type Conversion/1 -> Out1/1
  Sum of Elements/1 -> Data Type Conversion/1
  In1/1 -> Gain/1

== matlab function xmc_optical_flow/Moving Object/MATLAB Function ==
  data: z output; Angle parameter
function z = fcn(Angle)

coder.extrinsic('isSourceMovingObject')


persistent x;
persistent y;



shift_x = cos(Angle/180*pi);
shift_y = sin(Angle/180*pi);

if (isempty(x))
    x = 0; y = 0;
end

if ~isSourceMovingObject()
    x = 0; y = 0;
end

x = x+shift_x;
y = y+shift_y;

z = [1 0;
    0 1;
    x y];

== matlab function xmc_optical_flow/Flow Viewer/MATLAB Function1 ==
  data: gainValue output
function gainValue = fcn()
%#codegen
coder.extrinsic('getGainValue')

gainValue = 0;

gainValue = getGainValue();

== matlab function xmc_optical_flow/Flow Viewer/MATLAB Function ==
  data: u input; y output
function y = fcn(u)

y = ones(size(u));

== matlab function xmc_optical_flow/Flow Viewer/statistics ==
  data: mag input; ang input; mean output
function mean = fcn(mag,ang)

coder.extrinsic('updateHistogram')

weighted_mean = sum(sum(ang.*mag))/sum(sum(mag))/pi*180;


mean = weighted_mean;

updateHistogram(ang(mag~=0));
